simulink model "BicycleModel"  (R2022b)
settings: Solver=VariableStepAuto  StartTime=0.0  StopTime=5  RelTol=1e-3
model workspace: external: MATLAB File C:\Users\npn01\OneDrive - Mälardalens högskola\Desktop\Research\BPP\BicycleModelFillet\BicycleModelFillet_DataFile.m (data not in the file)
undefined symbols (not defined in the file or in its folder): pidParam, rndSeed, sigmaLean, sigmaSteer, smiData, Ts, TsInner, v, X, Y, Z
libraries: sm_lib x152, nesl_utility x8, simulink x2, simulink_extras x2, slpidlib x1, fl_lib x1
(part 4 of 4)

== matlab function BicycleModel/Bicycle/Sense/quaternion to euler ==
  data: q input; roll output; yaw output
function [roll,yaw] = fcn(q)

siny_cosp = 2*(q(1)*q(4) + q(2)*q(3));
cosy_cosp = 1 - 2*(q(3)*q(3) + q(4)*q(4));
yaw = atan2(siny_cosp,cosy_cosp) ;
%yaw = atan2(sin(yaw), cos(yaw));

sinr_cosp = 2 * (q(1) * q(2) + q(3) * q(4));
cosr_cosp = 1 - 2 * (q(2) * q(2) + q(3) * q(3));
roll=atan2(sinr_cosp, cosr_cosp);

%roll=roll+pi;
roll=atan2(sin(roll),cos(roll));
